simulink model "P2001_230206_CumulativeCostGD1"  (R2022b)
settings: Solver=VariableStepAuto  StartTime=0.0  StopTime=30  RelTol=1e-7
settings Model: Creator=turib  LastModifiedBy=turib

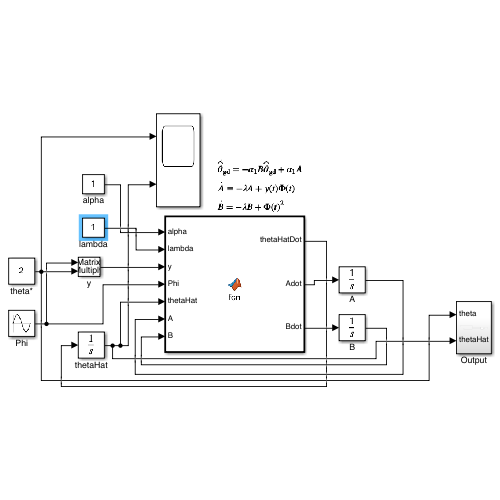
[thumbnail: Simulink's stored preview of the top-level diagram]
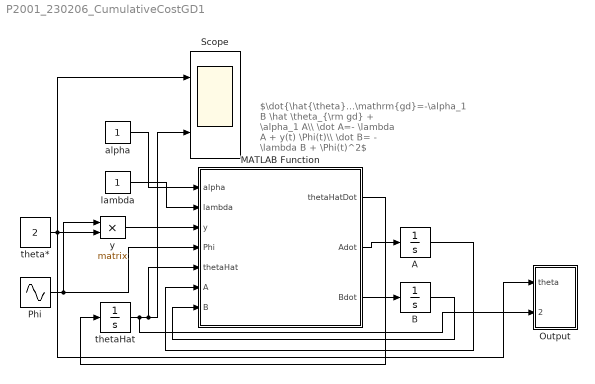
== system P2001_230206_CumulativeCostGD1 ==
  note: $\dot{\hat{\theta}}_\mathrm{gd}=-\alpha_1 B \hat \theta_{\rm gd} + \alpha_1 A\\ \dot A=- \lambda A + y(t) \Phi(t)\\ \dot B= - \lambda B + \Phi(t)^2$
  A : Integrator  InitialCondition=1
  B : Integrator  InitialCondition=1
  MATLAB Function : MATLAB Function  TreatAsAtomicUnit=on
  Output : Subsystem
  Phi : Sin  Frequency=2  Phase=1  SampleTime=0
  Scope : Scope  NumInputPorts=2
  alpha : Constant
  lambda : Constant
  theta* : Constant  Value=2
  thetaHat : Integrator
  y : Product  Multiplication=Matrix(*)  OutDataTypeStr=double
  wires:
  thetaHat/1 -> Output/2(thetaHat), Scope/2, MATLAB Function/5(thetaHat)
  A/1 -> MATLAB Function/6(A)
  theta*/1 -> Output/1(theta), Scope/1, y/2
  lambda/1 -> MATLAB Function/2(lambda)
  Phi/1 -> MATLAB Function/4(Phi), y/1
  alpha/1 -> MATLAB Function/1(alpha)
  y/1 -> MATLAB Function/3(y)
  MATLAB Function/1(thetaHatDot) -> thetaHat/1
  MATLAB Function/2(Adot) -> A/1
  MATLAB Function/3(Bdot) -> B/1
  B/1 -> MATLAB Function/7(B)

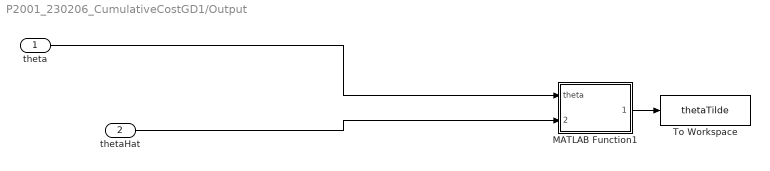
== system P2001_230206_CumulativeCostGD1/Output ==
  theta : Inport
  thetaHat : Inport  Port=2
  MATLAB Function1 : MATLAB Function  TreatAsAtomicUnit=on
  To Workspace : ToWorkspace  VariableName=thetaTilde  SampleTime=-1
  wires:
  MATLAB Function1/1(thetaTilde) -> To Workspace/1
  thetaHat/1 -> MATLAB Function1/2(thetaHat)
  theta/1 -> MATLAB Function1/1(theta)

== matlab function P2001_230206_CumulativeCostGD1/Output/MATLAB Function1 ==
  data: theta input; thetaTilde output; thetaHat input
function thetaTilde = error(theta, thetaHat)

thetaTilde = thetaHat - theta;

end

== matlab function P2001_230206_CumulativeCostGD1/MATLAB Function ==
  data: alpha input; thetaHatDot output; lambda input; Adot output; y input; Phi input; thetaHat input; A input; B input; Bdot output
function [thetaHatDot, Adot, Bdot] = fcn(alpha, lambda, y, Phi, ...
    thetaHat, A, B)

thetaHatDot = - alpha * B * thetaHat + alpha * A;
Adot = - lambda * A + y * Phi;
Bdot = - lambda * B + Phi ^ 2;

end
